simulink model "data_store_model_2019v"  (R2019b)
settings: Solver=VariableStepAuto  StartTime=0.0  StopTime=10.0  RelTol=1e-3
settings Model: Creator=Brigosha_Guest  LastModifiedBy=Brigosha_Guest
settings DebuggingCC: UnconnectedInputMsg=none  UnconnectedOutputMsg=none  UnconnectedLineMsg=none  SFMachineParentedDataDiag=error
settings ModelReferenceCC: EnableRefExpFcnMdlSchedulingChecks=off
settings RTWCC: Description=Generic Real-Time Target

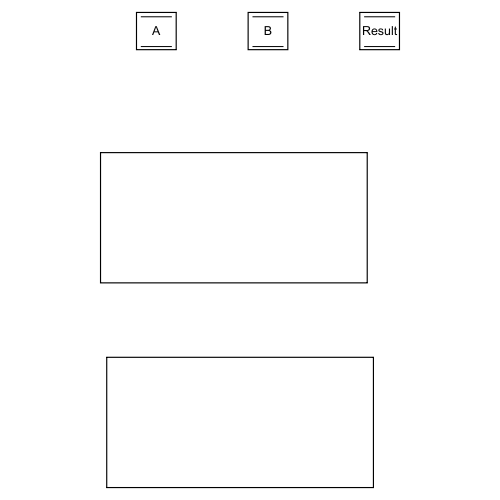
[thumbnail: Simulink's stored preview of the top-level diagram]
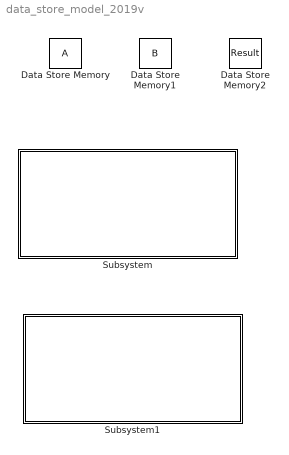
== system data_store_model_2019v ==
  Data Store Memory : DataStoreMemory  WriteAfterWriteMsg=warning  ShowAdditionalParam=off
  Data Store Memory1 : DataStoreMemory  DataStoreName=B  WriteAfterWriteMsg=warning  ShowAdditionalParam=off
  Data Store Memory2 : DataStoreMemory  DataStoreName=Result  WriteAfterWriteMsg=warning  ShowAdditionalParam=off
  Subsystem : Subsystem
  Subsystem1 : Subsystem

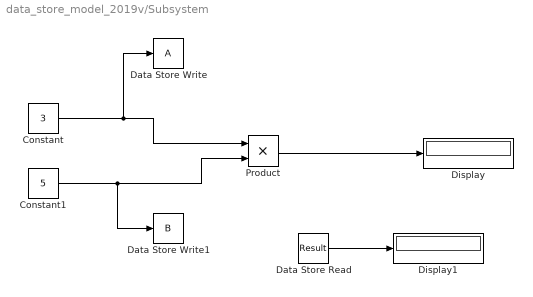
== system data_store_model_2019v/Subsystem ==
  Constant : Constant  Value=3
  Constant1 : Constant  Value=5
  Data Store Read : DataStoreRead  DataStoreName=Result
  Data Store Write : DataStoreWrite
  Data Store Write1 : DataStoreWrite  DataStoreName=B
  Display : Display
  Display1 : Display
  Product : Product
  wires:
  Constant1/1 -> Data Store Write1/1, Product/2
  Product/1 -> Display/1
  Constant/1 -> Data Store Write/1, Product/1
  Data Store Read/1 -> Display1/1

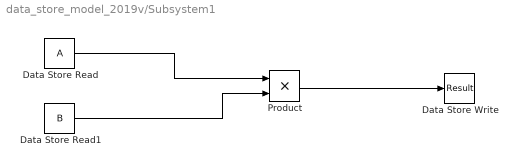
== system data_store_model_2019v/Subsystem1 ==
  Data Store Read : DataStoreRead
  Data Store Read1 : DataStoreRead  DataStoreName=B
  Data Store Write : DataStoreWrite  DataStoreName=Result
  Product : Product
  wires:
  Data Store Read/1 -> Product/1
  Product/1 -> Data Store Write/1
  Data Store Read1/1 -> Product/2
